simulink model "Simulink_fedic"  (R2022b)
settings: Solver=FixedStepDiscrete  StartTime=0.0  StopTime=2000  FixedStep=1  RelTol=1e-3
values from neighbouring files (symbols this model uses):
  coeff32 = zeros(16,1,'uint32')    [rom_dataconvert.m]
  stim = uint8(bin2dec(lines))    [tb_init.m]
libraries: hdlsllib x24, simulink x1
settings Model: PauseTimes=52  Creator=hamma  LastModifiedBy=hamma

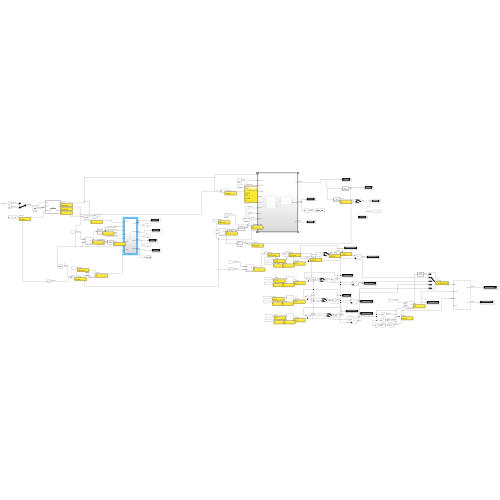
[thumbnail: Simulink's stored preview of the top-level diagram]
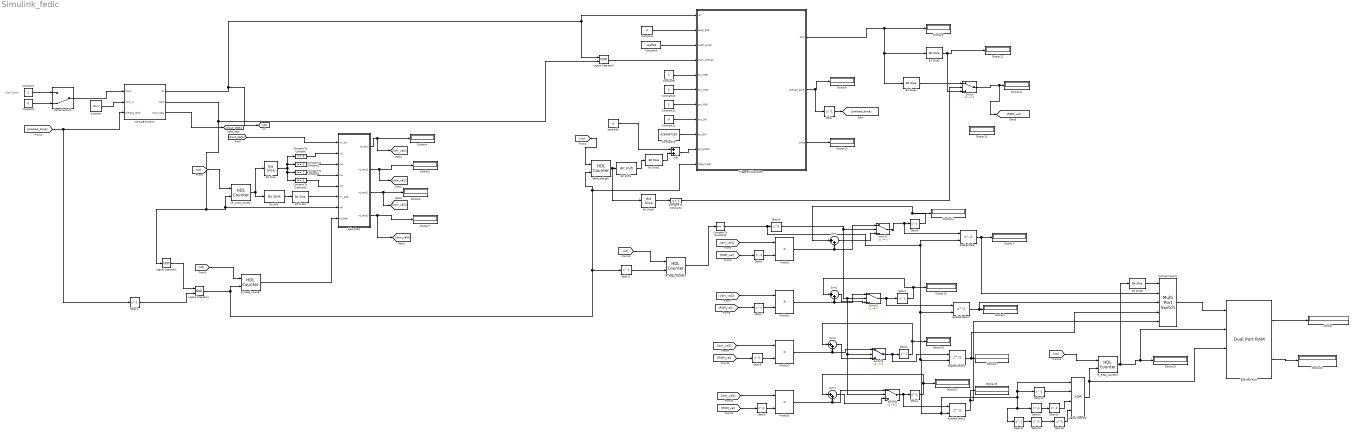
== system Simulink_fedic ==
  note: Start Signal
  Add : Sum
  Bit Shift : hdlsllib/Logic and Bit Operations/Bit Shift  mode=Shift Right Logical  N=2
  Bit Shift1 : hdlsllib/Logic and Bit Operations/Bit Shift  mode=Shift Right Logical  N=1
  Bit Slice : hdlsllib/Logic and Bit Operations/Bit Slice  lidx=1  ridx=0
  Bit Slice1 : hdlsllib/Logic and Bit Operations/Bit Slice  lidx=2  ridx=0
  Bit Slice2 : hdlsllib/Logic and Bit Operations/Bit Slice  lidx=3  ridx=0
  Bit Slice3 : hdlsllib/Logic and Bit Operations/Bit Slice  lidx=6  ridx=0
  Bit Slice4 : hdlsllib/Logic and Bit Operations/Bit Slice  lidx=13  ridx=7
  Bit Slice5 : hdlsllib/Logic and Bit Operations/Bit Slice  lidx=0  ridx=0
  Bit Slice6 : hdlsllib/Logic and Bit Operations/Bit Slice  lidx=1  ridx=0
  Compare To Constant : hdlsllib/Logic and Bit Operations/Compare To Constant  relop===  const=0  OutDataTypeStr=boolean
  Compare To Constant1 : hdlsllib/Logic and Bit Operations/Compare To Constant  relop===  const=1  OutDataTypeStr=boolean
  Compare To Constant2 : hdlsllib/Logic and Bit Operations/Compare To Constant  relop===  const=2  OutDataTypeStr=boolean
  Compare To Constant3 : hdlsllib/Logic and Bit Operations/Compare To Constant  relop===  const=3  OutDataTypeStr=boolean
  Compare To Constant4 : hdlsllib/Logic and Bit Operations/Compare To Constant  relop===  const=0  OutDataTypeStr=boolean
  Compare To Constant5 : simulink/Logic and Bit Operations/Compare To Constant  relop===  const=7  OutDataTypeStr=boolean
  Constant : Constant  Value=stim  VectorParams1D=off  SampleTime=-1
  Constant1 : Constant  OutDataTypeStr=boolean
  Constant10 : Constant  Value=0  OutDataTypeStr=boolean
  Constant11 : Constant  OutDataTypeStr=boolean
  Constant12 : Constant  Value=0  OutDataTypeStr=boolean
  Constant13 : Constant  Value=4294967295  VectorParams1D=off  OutDataTypeStr=uint32  SampleTime=-1
  Constant2 : Constant  Value=0  OutDataTypeStr=boolean
  Constant3 : Constant  Value=coeff32  VectorParams1D=off  OutDataTypeStr=uint32  SampleTime=-1
  Constant4 : Constant  Value=0  VectorParams1D=off  OutDataTypeStr=uint16  SampleTime=-1
  Constant9 : Constant  OutDataTypeStr=boolean
  Delay{,1..11,13..14,16,18..20} (18 alike) : Delay  DelayLength=1  InitialCondition=0
  Display{,1..20} (21 alike) : Display
  Dual Port RAM : hdlsllib/HDL RAMs/Dual Port RAM  ram_size=9
  Enabled Delay{,1..3} (4 alike) : Delay  DelayLength=1  ShowEnablePort=on
      settings: InputPortMap=u0,e6
  IR_Read_counter : hdlsllib/Sources/HDL Counter  CountType=Count limited  CountInit=0  CountStep=1  CountMax=7  CountFromType=Specify  CountFrom=0  CountResetPort=on  CountLoadPort=off  CountEnbPort=on  CountDirPort=off  CountHitOutputPort=off  CountDataType=Unsigned  CountWordLen=3  CountFracLen=0  CountSampTime=1
  IR_Read_counter1 : hdlsllib/Sources/HDL Counter  CountType=Count limited  CountInit=0  CountStep=1  CountMax=7  CountFromType=Initial value  CountFrom=0  CountResetPort=on  CountLoadPort=off  CountEnbPort=on  CountDirPort=off  CountHitOutputPort=off  CountDataType=Unsigned  CountWordLen=3  CountFracLen=0  CountSampTime=1
  IR_Read_counter2 : hdlsllib/Sources/HDL Counter  CountType=Count limited  CountInit=0  CountStep=1  CountMax=511  CountFromType=Initial value  CountFrom=0  CountResetPort=on  CountLoadPort=off  CountEnbPort=on  CountDirPort=off  CountHitOutputPort=off  CountDataType=Unsigned  CountWordLen=9  CountFracLen=0  CountSampTime=1
  IR_write_counter : hdlsllib/Sources/HDL Counter  CountType=Count limited  CountInit=0  CountStep=1  CountMax=31  CountFromType=Initial value  CountFrom=0  CountResetPort=on  CountLoadPort=off  CountEnbPort=on  CountDirPort=off  CountHitOutputPort=off  CountDataType=Unsigned  CountWordLen=5  CountFracLen=0  CountSampTime=1
  Logical Operator : Logic  Operator=XOR  Inputs=4  AllPortsSameDT=off  OutDataTypeStr=boolean
  Logical Operator1 : Logic  AllPortsSameDT=off  OutDataTypeStr=boolean
  Logical Operator2 : Logic  Operator=NOT  AllPortsSameDT=off  OutDataTypeStr=boolean
  Logical Operator5 : Logic  Operator=NOR  AllPortsSameDT=off  OutDataTypeStr=boolean
  MATLAB Function : MATLAB Function  TreatAsAtomicUnit=on
  Manual Switch2 : ManualSwitch  CurrentSetting=0
  Multiport Switch : MultiPortSwitch  DataPortOrder=Zero-based contiguous  Inputs=4  zeroidx=on  SaturateOnIntegerOverflow=off  InputSameDT=off
  Product : Product  OutDataTypeStr=uint32
  Product1 : Product  OutDataTypeStr=uint32  RndMeth=Nearest
  Product2 : Product  OutDataTypeStr=uint32
  Product3 : Product  OutDataTypeStr=uint32
  Subsystem : Subsystem
  Sum{,1..2,4} (4 alike) : Sum  Inputs=|++
  Switch{,1..4} (5 alike) : Switch  SaturateOnIntegerOverflow=off  InputSameDT=off
  Triggered Subsystem : Subsystem  TreatAsAtomicUnit=on
  base addr : Constant  Value=0  VectorParams1D=off  OutDataTypeStr=uint16  SampleTime=-1
  offset_add gen : hdlsllib/Sources/HDL Counter  CountType=Count limited  CountInit=0  CountStep=1  CountMax=31  CountFromType=Initial value  CountFrom=0  CountResetPort=on  CountLoadPort=off  CountEnbPort=on  CountDirPort=off  CountHitOutputPort=off  CountDataType=Unsigned  CountWordLen=5  CountFracLen=0  CountSampTime=1
  wires:
  Constant/1 -> MATLAB Function/2(stim_in)
  Constant1/1 -> Manual Switch2/1
  Manual Switch2/1 -> MATLAB Function/1(finish)
  Constant2/1 -> Manual Switch2/2
  MATLAB Function/3(input_data) -> [input_data]
  IR_write_counter/1 -> Bit Slice/1, Bit Shift/1
  [rst] -> IR_write_counter/1
  Bit Slice/1 -> Compare To Constant3/1, Compare To Constant2/1, Compare To Constant1/1, Compare To Constant/1
  MATLAB Function/2(start) -> Subsystem/7(In8), IR_write_counter/2, Logical Operator2/1, Logical Operator5/2
  Compare To Constant/1 -> Subsystem/2(In2)
  Compare To Constant1/1 -> Subsystem/3(In3)
  Compare To Constant2/1 -> Subsystem/4(In4)
  Compare To Constant3/1 -> Subsystem/5(In5)
  Bit Shift/1 -> Bit Slice1/1
  Subsystem/1(rd_dout) -> [ram_val1], Display4/1
  Subsystem/4(rd_dout3) -> [ram_val4], Display7/1
  Subsystem/3(rd_dout2) -> [ram_val3], Display6/1
  Subsystem/2(rd_dout1) -> [ram_val2], Display5/1
  Bit Slice1/1 -> Subsystem/6(wr_addr)
  [rst] -> IR_Read_counter/1
  Constant4/1 -> Triggered Subsystem/2(base_addr)
  Constant3/1 -> Triggered Subsystem/3(coeff_words)
  Logical Operator5/1 -> Triggered Subsystem/4(start_preload)
  [rst] -> offset_add gen/1
  Constant9/1 -> Triggered Subsystem/5(ext_MEN)
  Constant10/1 -> Triggered Subsystem/6(ext_WEN)
  Constant11/1 -> Triggered Subsystem/7(ext_REN)
  Constant12/1 -> Triggered Subsystem/8(ext_DIN)
  Constant13/1 -> Triggered Subsystem/9(ext_BM)
  Add/1 -> Triggered Subsystem/10(ext_ADDR)
  base addr/1 -> Add/1
  Triggered Subsystem/2(preload_done) -> Delay/1, Display9/1
  Triggered Subsystem/3(state) -> Display10/1
  MATLAB Function/1(rst) -> Triggered Subsystem/1(rst), Logical Operator5/1, [rst]
  Delay/1 -> [preload_done]
  Logical Operator2/1 -> Logical Operator1/1
  [preload_done] -> MATLAB Function/3(preload_done), Delay1/1
  Delay1/1 -> Logical Operator1/2
  Bit Shift1/1 -> Bit Slice2/1
  offset_add gen/1 -> Bit Slice5/1, Bit Shift1/1
  Bit Slice2/1 -> Add/2
  Bit Slice5/1 -> Compare To Constant4/1
  Compare To Constant4/1 -> Switch/2
  Bit Slice3/1 -> Switch/3, Display12/1
  Switch/1 -> [ROM_val], Display11/1
  Triggered Subsystem/1(dout) -> Bit Slice4/1, Bit Slice3/1, Display8/1
  Bit Slice4/1 -> Switch/1
  [ram_val1] -> Product/1
  [ROM_val] -> Delay5/1
  [ram_val2] -> Product1/1
  [ROM_val] -> Delay7/1
  [ROM_val] -> Delay8/1
  [ram_val4] -> Product3/1
  [ram_val3] -> Product2/1
  [ROM_val] -> Delay9/1
  Switch2/1 -> Enabled Delay1/1, Delay2/1
  Switch3/1 -> Enabled Delay2/1, Delay3/1
  IR_Read_counter/1 -> Subsystem/8(rd_addr)
  IR_Read_counter1/1 -> Compare To Constant5/1
  Product/1 -> Sum/2, Switch1/1
  Sum1/1 -> Switch2/3
  Product1/1 -> Switch2/1, Sum1/2
  Sum2/1 -> Switch3/3
  Product2/1 -> Switch3/1, Sum2/2
  Delay2/1 -> Sum1/1, Display15/1
  Delay3/1 -> Display16/1, Sum2/1
  Sum4/1 -> Switch4/3
  Delay4/1 -> Sum4/1, Display17/1
  Product3/1 -> Switch4/1, Sum4/2
  [rst] -> IR_Read_counter1/1
  Delay5/1 -> Product/2
  Delay7/1 -> Product1/2
  Delay8/1 -> Product2/2
  Delay9/1 -> Product3/2
  [input_data] -> Subsystem/1(wr_din)
  Logical Operator1/1 -> Delay11/1, Triggered Subsystem/11(read_mode), offset_add gen/2, IR_Read_counter/2
  Delay11/1 -> IR_Read_counter1/2
  Sum/1 -> Switch1/3
  Delay6/1 -> Display14/1, Sum/1
  Switch4/1 -> Enabled Delay3/1, Delay4/1
  Enabled Delay/1 -> Multiport Switch/2, Display1/1
  Enabled Delay1/1 -> Multiport Switch/3, Display2/1
  Enabled Delay2/1 -> Multiport Switch/4, Display3/1
  Enabled Delay3/1 -> Multiport Switch/5, Display18/1
  Delay10/1 -> Switch4/2, Switch3/2, Switch2/2, Switch1/2
  Switch1/1 -> Enabled Delay/1, Delay6/1
  [rst] -> IR_Read_counter2/1
  IR_Read_counter2/1 -> Dual Port RAM/2, Display19/1, Bit Slice6/1
  Delay13/1 -> Logical Operator/2
  Delay16/1 -> Delay14/1
  Delay14/1 -> Logical Operator/3
  Delay19/1 -> Delay18/1
  Delay20/1 -> Delay19/1
  Compare To Constant5/1 -> Enabled Delay2/2, Logical Operator/1, Delay13/1, Delay20/1, Delay16/1, Enabled Delay3/2, Enabled Delay1/2, Enabled Delay/2, Delay10/1
  Delay18/1 -> Logical Operator/4
  Logical Operator/1 -> IR_Read_counter2/2, Dual Port RAM/3
  Bit Slice6/1 -> Multiport Switch/1
  Multiport Switch/1 -> Dual Port RAM/1
  Dual Port RAM/1 -> Display/1
  Dual Port RAM/2 -> Display20/1

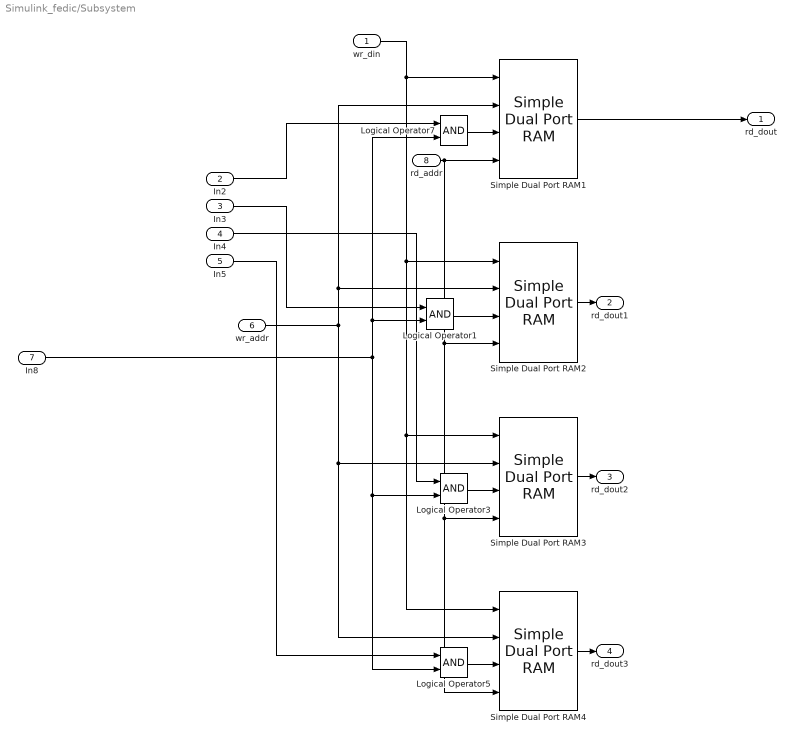
== system Simulink_fedic/Subsystem ==
  wr_din : Inport
  In2 : Inport  Port=2
  In3 : Inport  Port=3
  In4 : Inport  Port=4
  In5 : Inport  Port=5
  wr_addr : Inport  Port=6
  In8 : Inport  Port=7
  rd_addr : Inport  Port=8
  Logical Operator{1,3,5,7} (4 alike) : Logic  AllPortsSameDT=off  OutDataTypeStr=boolean
  Simple Dual Port RAM{1..4} (4 alike) : hdlsllib/HDL RAMs/Simple Dual Port RAM  ram_size=3
  rd_dout : Outport
  rd_dout1 : Outport  Port=2
  rd_dout2 : Outport  Port=3
  rd_dout3 : Outport  Port=4
  wires:
  In8/1 -> Logical Operator5/2, Logical Operator3/2, Logical Operator7/2, Logical Operator1/2
  In4/1 -> Logical Operator3/1
  rd_addr/1 -> Simple Dual Port RAM2/4, Simple Dual Port RAM3/4, Simple Dual Port RAM4/4, Simple Dual Port RAM1/4
  Simple Dual Port RAM3/1 -> rd_dout2/1
  Simple Dual Port RAM2/1 -> rd_dout1/1
  wr_din/1 -> Simple Dual Port RAM4/1, Simple Dual Port RAM3/1, Simple Dual Port RAM2/1, Simple Dual Port RAM1/1
  Logical Operator3/1 -> Simple Dual Port RAM3/3
  In5/1 -> Logical Operator5/1
  Logical Operator5/1 -> Simple Dual Port RAM4/3
  wr_addr/1 -> Simple Dual Port RAM4/2, Simple Dual Port RAM3/2, Simple Dual Port RAM2/2, Simple Dual Port RAM1/2
  Logical Operator1/1 -> Simple Dual Port RAM2/3
  Logical Operator7/1 -> Simple Dual Port RAM1/3
  Simple Dual Port RAM1/1 -> rd_dout/1
  In3/1 -> Logical Operator1/1
  Simple Dual Port RAM4/1 -> rd_dout3/1
  In2/1 -> Logical Operator7/1

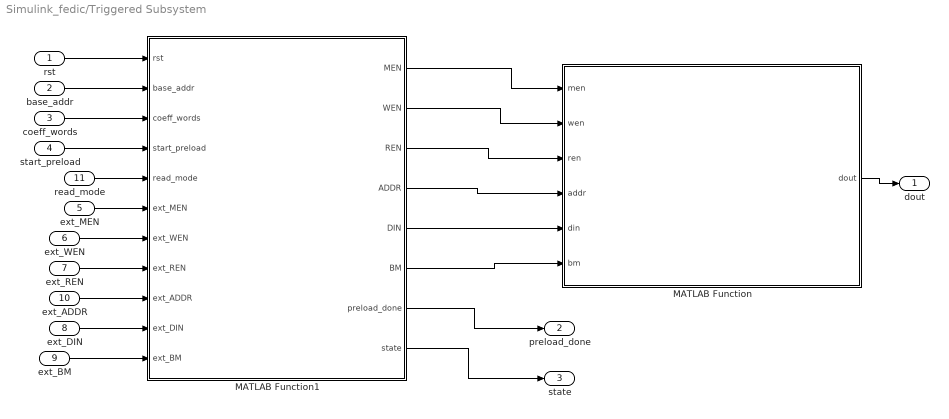
== system Simulink_fedic/Triggered Subsystem ==
  rst : Inport
  base_addr : Inport  Port=2
  coeff_words : Inport  Port=3
  start_preload : Inport  Port=4
  ext_MEN : Inport  Port=5
  ext_WEN : Inport  Port=6
  ext_REN : Inport  Port=7
  ext_DIN : Inport  Port=8
  ext_BM : Inport  Port=9
  ext_ADDR : Inport  Port=10
  read_mode : Inport  Port=11
  MATLAB Function : MATLAB Function  TreatAsAtomicUnit=on
  MATLAB Function1 : MATLAB Function  TreatAsAtomicUnit=on
  dout : Outport
  preload_done : Outport  Port=2  VectorParamsAs1DForOutWhenUnconnected=off
  state : Outport  Port=3  VectorParamsAs1DForOutWhenUnconnected=off
  wires:
  MATLAB Function/1(dout) -> dout/1
  MATLAB Function1/1(MEN) -> MATLAB Function/1(men)
  MATLAB Function1/2(WEN) -> MATLAB Function/2(wen)
  MATLAB Function1/3(REN) -> MATLAB Function/3(ren)
  MATLAB Function1/4(ADDR) -> MATLAB Function/4(addr)
  MATLAB Function1/5(DIN) -> MATLAB Function/5(din)
  MATLAB Function1/6(BM) -> MATLAB Function/6(bm)
  rst/1 -> MATLAB Function1/1(rst)
  base_addr/1 -> MATLAB Function1/2(base_addr)
  ext_BM/1 -> MATLAB Function1/11(ext_BM)
  ext_DIN/1 -> MATLAB Function1/10(ext_DIN)
  ext_ADDR/1 -> MATLAB Function1/9(ext_ADDR)
  ext_REN/1 -> MATLAB Function1/8(ext_REN)
  ext_WEN/1 -> MATLAB Function1/7(ext_WEN)
  ext_MEN/1 -> MATLAB Function1/6(ext_MEN)
  read_mode/1 -> MATLAB Function1/5(read_mode)
  start_preload/1 -> MATLAB Function1/4(start_preload)
  coeff_words/1 -> MATLAB Function1/3(coeff_words)
  MATLAB Function1/7(preload_done) -> preload_done/1
  MATLAB Function1/8(state) -> state/1

== matlab function Simulink_fedic/Triggered Subsystem/MATLAB Function ==
  data: men input; dout output; wen input; ren input; addr input; din input; bm input
function dout  = sram_step(men, wen, ren, addr, din, bm)
persistent mem dr
if isempty(mem)
    mem = zeros(512,1,'uint32');   % EXACT: 512 words
    dr  = uint32(0);               % EXACT: 32-bit output reg
end

if men
    if wen
        old = mem(double(addr)+1);
        new = bitor(bitand(old, bitcmp(uint32(bm))), bitand(uint32(din), uint32(bm)));
        mem(double(addr)+1) = new;
        if ren
            dr = new; % write-through
        end
    elseif ren
        dr = mem(double(addr)+1); % synchronous read (registered)
    end
end

dout = dr;

== matlab function Simulink_fedic/MATLAB Function ==
  data: finish input; rst output; stim_in input; start output; input_data output; preload_done input
function [rst, start, input_data] = TB_Generator(finish, stim_in, preload_done)
%#codegen
RESET_CYCLES = uint16(5);
SAMPLES_PER_MATRIX = uint16(32);

% States:
% 0=RESET_HOLD, 1=WAIT_PRELOAD, 2=STREAM, 3=WAIT_FINISH
persistent state reset_cnt matrix_idx sample_idx finish_d

if isempty(state)
    state = uint8(0);
    reset_cnt  = uint16(0);
    matrix_idx = uint16(0);
    sample_idx = uint16(0);
    finish_d   = false;
end

% Default outputs
rst = false;
start = false;
input_data = uint8(0);

% Detect finish rising edge
finish_rise = (finish && ~finish_d);
finish_d = finish;

switch state
    % ----------------------------
    case uint8(0)  % RESET_HOLD (5 cycles)
        rst = true;
        start = false;
        input_data = uint8(0);

        if reset_cnt == RESET_CYCLES-1
            rst = false;                 % deassert after 5th cycle
            state = uint8(1);            % go wait preload
        else
            reset_cnt = reset_cnt + 1;
        end

    % ----------------------------
    case uint8(1)  % WAIT_PRELOAD
        rst = false;
        start = false;
        input_data = uint8(0);

        if preload_done
            % Start streaming first matrix
            sample_idx = uint16(0);
            state = uint8(2); % STREAM
        end

    % ----------------------------
    case uint8(2)  % STREAM 32 samples
        rst = false;
        start = true;

        addr = matrix_idx * SAMPLES_PER_MATRIX + sample_idx; % 0-based
        idx  = addr + 1; % MATLAB indexing

        if idx >= 1 && idx <= uint16(2048)
            input_data = stim_in(idx);
        else
            input_data = uint8(0);
        end

        if sample_idx == SAMPLES_PER_MATRIX-1
            state = uint8(3);  % WAIT_FINISH
        else
            sample_idx = sample_idx + 1;
        end

    % ----------------------------
    otherwise  % WAIT_FINISH
        rst = false;
        start = false;
        input_data = uint8(0);

        if finish_rise
            matrix_idx = matrix_idx + 1;
            sample_idx = uint16(0);
            state = uint8(2); % STREAM next matrix
        end
end
end

== matlab function Simulink_fedic/Triggered Subsystem/MATLAB Function1 ==
  data: rst input; MEN output; base_addr input; coeff_words input; WEN output; REN output; ADDR output; DIN output; BM output; preload_done output; start_preload input; read_mode input; ext_MEN input; ext_WEN input; ext_REN input; ext_ADDR input; ext_DIN input; ext_BM input; state output
function [MEN,WEN,REN,ADDR,DIN,BM, preload_done, state] = ...
    rom_pin_mux_ctrl(rst, base_addr, coeff_words, start_preload, ...
                     read_mode, ext_MEN, ext_WEN, ext_REN, ext_ADDR, ext_DIN, ext_BM)
%#codegen
persistent st idx done
if isempty(st)
    st   = uint8(0);   % 0=IDLE,1=PRELOAD,2=READ_PASS
    idx  = uint16(0);
    done = false;      % this is preload_done latch
end

N = uint16(numel(coeff_words));

% Defaults (idle)
MEN  = false; WEN = false; REN = false;
ADDR = uint16(base_addr);
DIN  = uint32(0);
BM   = uint32(hex2dec('FFFFFFFF'));

% Reset clears preload_done
if rst
    st   = uint8(0);
    idx  = uint16(0);
    done = false;
    preload_done = done;
    state = st;
    return;
end

% READ pass-through priority
if read_mode
    st = uint8(2);

    MEN  = logical(ext_MEN);
    WEN  = logical(ext_WEN);
    REN  = logical(ext_REN);
    ADDR = uint16(ext_ADDR);
    DIN  = uint32(ext_DIN);
    BM   = uint32(ext_BM);

    preload_done = done;
    state = st;
    return;
end

% Internal preload/idle
switch st
    case uint8(0)  % IDLE
        % only start preload if not already done
        if start_preload && ~done
            st  = uint8(1);   % PRELOAD
            idx = uint16(0);
        end

    case uint8(1)  % PRELOAD
        MEN = true;
        WEN = true;
        REN = false;

        ADDR = uint16(base_addr + idx);
        DIN  = uint32(coeff_words(double(idx)+1));

        if idx == (N-1)
            done = true;       % latch stays high until reset
            st   = uint8(0);   % back to IDLE
        else
            idx = idx + 1;
        end

    otherwise
        st = uint8(0);
end

preload_done = done;
state = st;
end
